simulink model "modelo_ideal_Practica3"  (R2021a)
settings: Solver=VariableStepAuto  StartTime=0.0  StopTime=10.0  MaxStep=1e-5  RelTol=1e-3
values from neighbouring files (symbols this model uses):
  k_e = 132500    [modelo_ideal_Practica6.mat]    (also in modelo_ideal_practica3_workspace.mat; modelo_practica4_workspace.mat; modelo_real_practica5_workspace.mat)
  p = 125.59    [modelo_ideal_Practica6.mat]    (also in modelo_ideal_practica3_workspace.mat; modelo_practica4_workspace.mat; modelo_real_practica5_workspace.mat)
  T = 0.005    [modelo_ideal_Practica6.mat]    (also in modelo_ideal_practica3_workspace.mat = 0.001; modelo_real_practica5_workspace.mat)
  Vmax = 12    [modelo_ideal_practica3_workspace.mat]
libraries: simulink x2
settings Model: Creator=Marcial  LastModifiedBy=Marcial

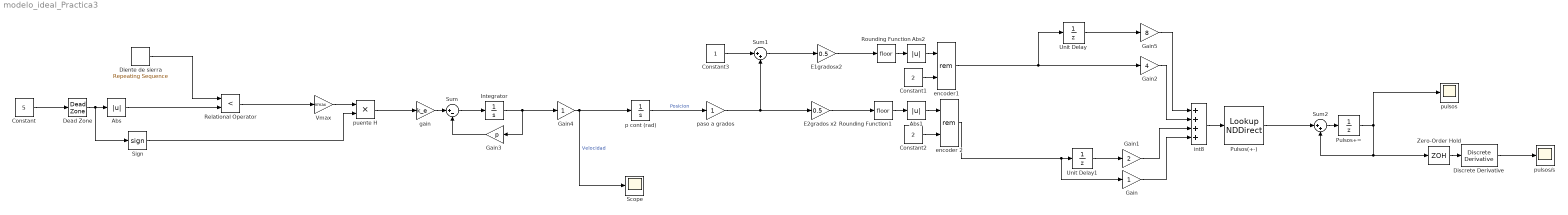
== system modelo_ideal_Practica3 ==
  Abs : Abs
  Abs1 : Abs
  Abs2 : Abs
  Constant : Constant  Value=5
  Constant1 : Constant  Value=2
  Constant2 : Constant  Value=2
  Constant3 : Constant
  Dead Zone : DeadZone  SaturateOnIntegerOverflow=on
  Diente de sierra : simulink/Sources/Repeating Sequence  rep_seq_t=linspace(0,T,100)  rep_seq_y=linspace(0,Vmax,100)
  Discrete Derivative : simulink/Discrete/Discrete Derivative  gainval=1.0  ICPrevScaledInput=0.0  OutMin=[]  OutMax=[]  OutDataType=fixdt(1, 16)  OutScaling=2^-10  DoSatur=off
  E1gradosx2 : Gain  Gain=0.5
  E2grados x2 : Gain  Gain=0.5
  Gain : Gain
  Gain1 : Gain  Gain=2
  Gain2 : Gain  Gain=4
  Gain3 : Gain  Gain=p
  Gain4 : Gain
  Gain5 : Gain  Gain=8
  Integrator : Integrator
  Pulsos(+-) : LookupNDDirect  NumberOfTableDimensions=1  Table=[0,-1,1,0,1,0,0,-1,-1,0,0,1,0,1,-1,0];
  Pulsos+= : UnitDelay  SampleTime=-1  HasFrameUpgradeWarning=on
  Relational Operator : RelationalOperator  Operator=<  OutDataTypeStr=boolean  RndMeth=Simplest
  Rounding Function : Rounding
  Rounding Function1 : Rounding
  Scope : Scope
  Sign : Signum
  Sum : Sum  Inputs=|+-
  Sum1 : Sum  Inputs=|++
  Sum2 : Sum  Inputs=|++
  Unit Delay : UnitDelay  SampleTime=0.0001  HasFrameUpgradeWarning=on
  Unit Delay1 : UnitDelay  SampleTime=0.0001  HasFrameUpgradeWarning=on
  Vmax : Gain  Gain=Vmax
  Zero-Order Hold : ZeroOrderHold
  encoder 2 : Math  Operator=rem  SignedPower=on  SaturateOnIntegerOverflow=on
  encoder1 : Math  Operator=rem  SignedPower=on  SaturateOnIntegerOverflow=on
  gain : Gain  Gain=k_e
  int8 : Sum  Inputs=++++
  p cont (rad) : Integrator
  paso a grados : Gain
  puente H : Product
  pulsos : Scope
  pulsos/s : Scope
  wires:
  Dead Zone/1 -> Sign/1, Abs/1
  Sign/1 -> puente H/2
  Constant/1 -> Dead Zone/1
  Gain4/1 -> Scope/1, p cont (rad)/1  "Velocidad"
  Vmax/1 -> puente H/1
  Abs/1 -> Relational Operator/2
  Diente de sierra/1 -> Relational Operator/1
  Relational Operator/1 -> Vmax/1
  gain/1 -> Sum/1
  Gain3/1 -> Sum/2
  puente H/1 -> gain/1
  Integrator/1 -> Gain3/1, Gain4/1
  Sum/1 -> Integrator/1
  Abs1/1 -> encoder 2/1
  Abs2/1 -> encoder1/1
  Rounding Function/1 -> Abs2/1
  paso a grados/1 -> E2grados x2/1, Sum1/2
  Constant2/1 -> encoder 2/2
  E2grados x2/1 -> Rounding Function1/1
  Constant1/1 -> encoder1/2
  E1gradosx2/1 -> Rounding Function/1
  Sum1/1 -> E1gradosx2/1
  Rounding Function1/1 -> Abs1/1
  Constant3/1 -> Sum1/1
  p cont (rad)/1 -> paso a grados/1  "Posicion"
  Zero-Order Hold/1 -> Discrete Derivative/1
  Pulsos(+-)/1 -> Sum2/1
  Gain5/1 -> int8/1
  int8/1 -> Pulsos(+-)/1
  Sum2/1 -> Pulsos+=/1
  Pulsos+=/1 -> Zero-Order Hold/1, Sum2/2, pulsos/1
  encoder 2/1 -> Gain/1, Unit Delay1/1
  Gain1/1 -> int8/3
  Unit Delay/1 -> Gain5/1
  encoder1/1 -> Unit Delay/1, Gain2/1
  Gain2/1 -> int8/2
  Discrete Derivative/1 -> pulsos/s/1
  Gain/1 -> int8/4
  Unit Delay1/1 -> Gain1/1
